simulink model "exampleMinRunTime"  (Simulink 7.6)
settings: Solver=ode45  StartTime=0.0  StopTime=30  RelTol=1e-3
settings Model: Creator=drhf  LastModifiedBy=awohlfei
settings CodeAppCC: CustomSymbolStrType=$N$R$M_T

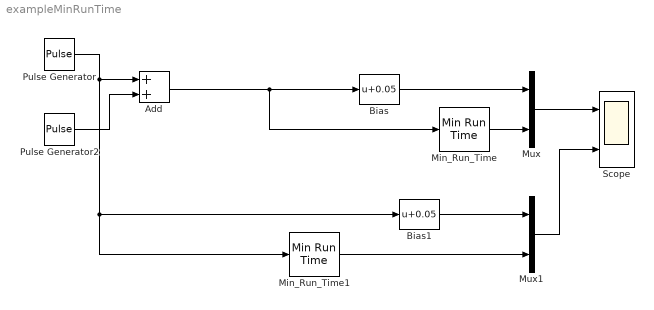
== system exampleMinRunTime ==
  Add : Sum
  Bias : Bias  Bias=0.05
  Bias1 : Bias  Bias=0.05
  Min_Run_Time : Reference  SystemSampleTime=-1  tminrun=2  mv=2
  Min_Run_Time1 : Reference  SystemSampleTime=-1  tminrun=5  mv=0.5
  Mux : Mux  Inputs=2
  Mux1 : Mux  Inputs=2
  Pulse Generator : DiscretePulseGenerator  PulseType=Time based  Period=10  PulseWidth=5
  Pulse Generator2 : DiscretePulseGenerator  PulseType=Time based  Period=20  PulseWidth=60
  Scope : Scope  NumInputPorts=2
      settings: YMin=-5~-5  YMax=5~5
  wires:
  Add/1 -> Min_Run_Time/1, Bias/1
  Mux/1 -> Scope/1
  Min_Run_Time/1 -> Mux/2
  Min_Run_Time1/1 -> Mux1/2
  Mux1/1 -> Scope/2
  Pulse Generator/1 -> Add/1, Bias1/1, Min_Run_Time1/1
  Pulse Generator2/1 -> Add/2
  Bias/1 -> Mux/1
  Bias1/1 -> Mux1/1
